simulink model "SSN_39busRT_Ctrl_4WT_19B"  (R2021a)
settings: Solver=ode3  StartTime=0.0  StopTime=10  FixedStep=Ts  MaxStep=1/60  RelTol=1e-2  AbsTol=1e-1
PreLoadFcn:
  | Ts=2.50e-6; ssn_ieee39_params; load('Pwf.mat');
InitFcn:
  | Ts=2.50e-6; ssn_ieee39_params; load('Pwf.mat');
values from neighbouring files (symbols this model uses):
  f = 50    [ssn_ieee39_params_ctrl.m]
  fNom = f    (= 60)    [ssn_ieee39_params_ctrl.m]
  ILR = 5.02    [ssn_ieee39_params_ctrl.m]
  IQMIN = 0.1    [ssn_ieee39_params_ctrl.m]
  ISCLIM = 1    [ssn_ieee39_params_ctrl.m]
  ITFpu = 1.10    (= 1.1)    [ssn_ieee39_params_ctrl.m]
  K = 1    [ssn_ieee39_params_ctrl.m]
  K1 = 1    [ssn_ieee39_params_ctrl.m]
  K2 = 2    [ssn_ieee39_params_ctrl.m]
  KCL = 1.04    [ssn_ieee39_params_ctrl.m]
  KFB = 0    [ssn_ieee39_params_ctrl.m]
  KFF = 1    [ssn_ieee39_params_ctrl.m]
  KFIX = 1    [ssn_ieee39_params_ctrl.m]
  KG = 1    [ssn_ieee39_params_ctrl.m]
  KIA = 59.91    [ssn_ieee39_params_ctrl.m]
  KIOEX = 0.0303    [ssn_ieee39_params_ctrl.m]
  KIUEX = 0.0303    [ssn_ieee39_params_ctrl.m]
  KIUOEX = 1    [ssn_ieee39_params_ctrl.m]
  KIUUEX = 1    [ssn_ieee39_params_ctrl.m]
  KLR = 22.47    [ssn_ieee39_params_ctrl.m]
  KM = 1    [ssn_ieee39_params_ctrl.m]
  KOEL = 0.24    [ssn_ieee39_params_ctrl.m]
  Kp = 1    [ssn_ieee39_params_ctrl.m]
  KPA = 30    [ssn_ieee39_params_ctrl.m]
  KPOEL = 1    [ssn_ieee39_params_ctrl.m]
  KPOEX = 0    [ssn_ieee39_params_ctrl.m]
  KPUEX = 0    [ssn_ieee39_params_ctrl.m]
  KSCALE = 0.319    [ssn_ieee39_params_ctrl.m]
  KUF = 0    [ssn_ieee39_params_ctrl.m]
  KUI = 0.001    [ssn_ieee39_params_ctrl.m]
  KUL = 0.24    [ssn_ieee39_params_ctrl.m]
  s = 10    [ssn_ieee39_params_ctrl.m]
  TA = 0.01    [ssn_ieee39_params_ctrl.m]
  Tadj = 0    [ssn_ieee39_params_ctrl.m]
  taps = [1 1 1.07 1.07 1.009 1.025 1 1.025 1.025 1.025]*1    [ssn_ieee39_params_ctrl.m]
  TF = 0.02    [ssn_ieee39_params_ctrl.m]
  TG = 0.024    [ssn_ieee39_params_ctrl.m]
  TINV = 0    [ssn_ieee39_params_ctrl.m]
  TIT = 0.1    [ssn_ieee39_params_ctrl.m]
  TL_10_11_len = 14    [ssn_ieee39_params_ctrl.m]
  TL_10_13_len = 14    [ssn_ieee39_params_ctrl.m]
  TL_13_14_len = 32    [ssn_ieee39_params_ctrl.m]
  TL_14_15_len = 70    [ssn_ieee39_params_ctrl.m]
  TL_15_16_len = 31.5    [ssn_ieee39_params_ctrl.m]
  TL_16_17_len = 26    [ssn_ieee39_params_ctrl.m]
  TL_16_19_len = 61    [ssn_ieee39_params_ctrl.m]
  TL_16_21_len = 46    [ssn_ieee39_params_ctrl.m]
  TL_16_24_len = 15    [ssn_ieee39_params_ctrl.m]
  TL_17_18_len = 26    [ssn_ieee39_params_ctrl.m]
  TL_17_27_len = 59    [ssn_ieee39_params_ctrl.m]
  TL_1_2_len = 134    [ssn_ieee39_params_ctrl.m]
  TL_1_39_len = 105    [ssn_ieee39_params_ctrl.m]
  TL_21_22_len = 47    [ssn_ieee39_params_ctrl.m]
  TL_22_23_len = 33    [ssn_ieee39_params_ctrl.m]
  TL_24_23_len = 88    [ssn_ieee39_params_ctrl.m]
  TL_25_26_len = 101    [ssn_ieee39_params_ctrl.m]
  TL_26_27_len = 46.5    [ssn_ieee39_params_ctrl.m]
  TL_26_28_len = 151    [ssn_ieee39_params_ctrl.m]
  TL_26_29_len = 200    [ssn_ieee39_params_ctrl.m]
  TL_28_29_len = 48    [ssn_ieee39_params_ctrl.m]
  TL_2_25_len = 28    [ssn_ieee39_params_ctrl.m]
  TL_2_2_len = 49    [ssn_ieee39_params_ctrl.m]
  TL_3_18_len = 42    [ssn_ieee39_params_ctrl.m]
  TL_3_4_len = 53    [ssn_ieee39_params_ctrl.m]
  TL_4_14_len = 33    [ssn_ieee39_params_ctrl.m]
  TL_4_5_len = 32.5    [ssn_ieee39_params_ctrl.m]
  TL_5_6_len = 14    [ssn_ieee39_params_ctrl.m]
  TL_5_8_len = 32    [ssn_ieee39_params_ctrl.m]
  TL_6_11_len = 26.5    [ssn_ieee39_params_ctrl.m]
  TL_6_7_len = 25.5    [ssn_ieee39_params_ctrl.m]
  TL_7_8_len = 15    [ssn_ieee39_params_ctrl.m]
  TL_8_9_len = 93    [ssn_ieee39_params_ctrl.m]
  TL_9_39_len = 136    [ssn_ieee39_params_ctrl.m]
  TOEL = 5.00    (= 5)    [ssn_ieee39_params_ctrl.m]
  TQREF = 0    [ssn_ieee39_params_ctrl.m]
  TQSCL = 0.012    [ssn_ieee39_params_ctrl.m]
  Ts_PMU = 1/1000    (= 0.001)    [ssn_ieee39_params_ctrl.m]
  TU1 = 0    [ssn_ieee39_params_ctrl.m]
  TU2 = 0    [ssn_ieee39_params_ctrl.m]
  TU3 = 0    [ssn_ieee39_params_ctrl.m]
  TU4 = 0    [ssn_ieee39_params_ctrl.m]
  TUL = 0    [ssn_ieee39_params_ctrl.m]
  TUP = 0.050    (= 0.05)    [ssn_ieee39_params_ctrl.m]
  TUQ = .005    (= 0.005)    [ssn_ieee39_params_ctrl.m]
  TUV = 0.2    [ssn_ieee39_params_ctrl.m]
  VAAMAX = VAMAX    (= 7.05)    [ssn_ieee39_params_ctrl.m]
  VAMAX = 7.05    [ssn_ieee39_params_ctrl.m]
  VAMIN = -6.11    [ssn_ieee39_params_ctrl.m]
  VBMAX = 999    [ssn_ieee39_params_ctrl.m]
  VF = 0    [ssn_ieee39_params_ctrl.m]
  VFB = 0    [ssn_ieee39_params_ctrl.m]
  VMMAX = 7.05    [ssn_ieee39_params_ctrl.m]
  VMMIN = -6.11    [ssn_ieee39_params_ctrl.m]
  VOELmax1 = 0.2353    [ssn_ieee39_params_ctrl.m]
  VOELmax2 = 0.0    (= 0)    [ssn_ieee39_params_ctrl.m]
  VOELmin1 = -0.24    [ssn_ieee39_params_ctrl.m]
  VOELmin2 = -1.0    (= -1)    [ssn_ieee39_params_ctrl.m]
  VRMAX = 7.05    [ssn_ieee39_params_ctrl.m]
  VRMIN = -6.11    [ssn_ieee39_params_ctrl.m]
  VSCLmax = 0.20    (= 0.2)    [ssn_ieee39_params_ctrl.m]
  VSCLmin = -0.10    (= -0.1)    [ssn_ieee39_params_ctrl.m]
  VUELmax1 = 1    [ssn_ieee39_params_ctrl.m]
  VUELmax2 = 1    [ssn_ieee39_params_ctrl.m]
  VUELmin1 = -1    [ssn_ieee39_params_ctrl.m]
  VUELmin2 = -1    [ssn_ieee39_params_ctrl.m]
  VUImax = 1    [ssn_ieee39_params_ctrl.m]
  VUImin = -1    [ssn_ieee39_params_ctrl.m]
undefined symbols (not defined in the file or in its folder): another_event_name, D1, Delta, DiscIntNeverNeededParam, find_system, MOV_segment9, my_event_name, powergui, Pw1, Pw2, Pw3, Pw4, vNomHV
libraries: powerlib_extras x162, spsThreePhaseVIMeasurementLib x55, spsCurrentMeasurementLib x52, simulink_extras x44, slpidlib x40, op_dpl_lib x36, spsST2AModel x20, spsThreePhaseParallelRLCLoadLib x20, spsThreePhaseTransformerTwoWindingsLib x17, spsControlledVoltageSourceLib x16, spsVoltageMeasurementLib x12, spsSynchronousMachinepuStandardLib x10
(part 14 of 19)

== system SSN_39busRT_Ctrl_4WT_19B/SM_master/4 WT/SS_windfarm3to4/Wind Farm (DFIG Type)/Wind Turbine Doubly-Fed Induction Generator (Average Model)1 ==
  Wind Power : Inport
  Asynchronous Machine pu Units1 : spsAsynchronousMachinepuUnitsLib/Asynchronous Machine pu Units  RotorType=Wound  PresetModel=No  MechanicalLoad=Torque Tm  ShowDetailedParameters=on  ReferenceFrame=Rotor  Units=pu  MeasurementBus=off  NominalParameters=[ Pnom*NumberOfUnits Vnom Fnom ]  VoltageRatio=1  Stator=[ Rs Lls]  Rotor=[ Rr Llr]  Cage1=[0.01909 0.0397]  Cage2=[0.01909 0.0397]  Lm=Lm  Mechanical=[H F p]  PolePairs=3  InitialConditions=[-4.81362e-32 0 0.00115467 0.00115467 0.00115467 -120.432 119.568 -0.43182]  SimulateSaturation=off  Saturation="[0.212,0.4201,0.8125,1.0979,1.4799,2.2457,3.2586,4.5763,6.4763 ;   0.5,0.7,0.9,1,1.1,1.2 ,1.3,1.4,1.5]"  LoadFlowParameters=0  TsPowergui=0  TsBlock=-1  IterativeModel=Forward Euler  IterativeDiscreteModel=Trapezoidal non iterative  Pmec=0
      settings: SourceProductBaseCode=PS
  Average_VSC : Subsystem  mask(Average Voltage Source converter){Ts=Ts_Power}
      mask prompts: Ts "Sample time"
  Average_VSC1 : Subsystem  mask(Average Voltage Source converter){Ts=Ts_Power}
      mask prompts: Ts "Sample time"
  B1 : spsThreePhaseVIMeasurementLib/Three-Phase V-I Measurement  VoltageMeasurement=phase-to-ground  SetLabelV=off  LabelV=Vabc_B1  Vpu=on  VpuLL=off  CurrentMeasurement=yes  SetLabelI=off  LabelI=Iabc_Beol  Ipu=on  Pbase=Pnom*NumberOfUnits  Vbase=Vnom  OutputType=Complex  PhasorSimulation=off  PSBequivalent=0
  Bus Selector : BusSelector  OutputSignals=Mechanical.Rotor speed (wm),Mechanical.Rotor angle thetam (rad),Mechanical.Electromagnetic torque Te (pu)
  C2 : spsSeriesRLCBranchLib/Series RLC Branch  LConnTagsString=__new0  RConnTagsString=__new0  BranchType=C  Resistance=1.0  Inductance=1.0  SetiL0=off  InitialCurrent=0  Capacitance=C_DClink*NumberOfUnits  Setx0=off  InitialVoltage=0  Measurements=Branch voltage
  Control System_average : Subsystem  mask{Pmax=0.5, Vdc_nom=Vdc_nom*1.2, capacitor=C_DClink*NumberOfUnits, speed_ABCD=[0.7 0.71 1.2 1.21], power_C=power_C, pitch_gain=500, pitch_max=45, pitch_rate=2, Kpi_Q=[0.05 5], Kpi_dc_reg=[0.002 0.05], Kpi_grid_side_cur_reg=[2.5 500], Kpi_rotor_side_cur_reg=[0.3 8], Q_slew_rate=100, torque_slew_rate=1, current_slew_rate=200, Ts=Ts_Power, Ts_Control=Ts_Control}
      mask prompts: Pmax "Converter maximum power (p.u.):"; Vdc_nom "Nominal DC bus voltage (V):"; capacitor "DC bus capacitor (F):"; speed_ABCD "Tracking characteristic speeds: [speed_A(pu) ... speed_D(pu)]"; power_C "Power at point C (pu/mechanical power):"; pitch_gain "Pitch angle controller gain [Kp]:"; pitch_max "Maximum pitch angle (deg):"; pitch_rate "Maximum rate of change of pitch angle (deg/s):"; Kpi_Q "Reactive power regulator gains: [Kp Ki]"; Kpi_dc_reg "DC bus voltage regulator gains: [Kp Ki]"; Kpi_grid_side_cur_reg "Grid-side converter current regulator gains: [Kp Ki]"; Kpi_rotor_side_cur_reg "Rotor-side converter current regulator gains: [Kp Ki]"; Q_slew_rate "Maximum rate of change of reference reactive power (p.u./s):"; torque_slew_rate "Maximum rate of change of reference torque (p.u./s):"; current_slew_rate "Maximum rate of change of converter  reference currents (p.u./s):"; Ts "Sample time"; Ts_Control "Sample time control"
      mask init: same as SSN_39busRT_Ctrl_4WT_19B/SM_master/4 WT/SS_windfarm1to2/Wind Farm (DFIG Type)/Wind Turbine Doubly-Fed Induction Generator (Average Model)1/Control System_average
  Data acquisition electrical : Subsystem
  "Iq_ref (pu) " : Constant  Value=0
  "Qref (pu) " : Constant  Value=0
  Subsystem : Subsystem
  Subsystem1 : Subsystem
  Subsystem2 : Subsystem
  Vc1 : spsVoltageMeasurementLib/Voltage Measurement  PhasorSimulation=off  OutputType=Complex  PSBequivalent=0
  Wind Turbine v : Subsystem  mask{Pnom=Pmec*NumberOfUnits, Pelec_base=Pnom*NumberOfUnits, wind_base=11, P_wind_base=power_C, speed_nom=speed_C, pitch_angle=0, c1_c6=[0.51763          116          0.4            5           21     0.006795], cp_nom=0.48, lambda_nom=8.1}
      mask prompts: Pnom "Nominal mechanical output power(W):"; Pelec_base "Base power of the electrical genera(VA):"; wind_base "Base wind speed(m/s):"; P_wind_base "Maximum powe at base wind speed(pu of nominal mechanical power):"; speed_nom "Base rotational speed(p.u. of base generator speed):"; pitch_angle "Pitch angle beta to display wind-turbine power"
      mask init:
      | c1=c1_c6(1);c2=c1_c6(2);c3=c1_c6(3);c4=c1_c6(4);c5=c1_c6(5);c6=c1_c6(6);
      | power_initmask();
      mask DialogControl DisplayTurbChar Prompt: Display wind turbine power characteristics
      mask DialogControl DisplayTurbChar Callback: WindTurbinePlot(gcb)
  "choke " : spsThreePhaseSeriesRLCBranchLib/Three-Phase Series RLC Branch  LConnTagsString=A|B|C  RConnTagsString=A|B|C  BranchType=RL  Resistance=R_RL*Vnom^2/(Pnom*NumberOfUnits)  Inductance=L_RL*Vnom^2/(Pnom*NumberOfUnits)/(2*pi*Fnom)  Capacitance=1.0  Measurements=None
  A : PMIOPort  Side=Left
  B : PMIOPort  Port=2  Side=Left
  C : PMIOPort  Port=3  Side=Left
  meas_elec : Outport
  wires:
  "Iq_ref (pu) "/1 -> Control System_average/3(Iq_grid_conv_ref)
  "Qref (pu) "/1 -> Control System_average/2(Q_ref)
  [Vabc_B1] -> Control System_average/1(Vabc_B1)
  B1/1 -> [Vabc_B1]
  B1/2 -> [Iabc_B1]
  Subsystem2/1(IabcPU) -> [Iabc_stator]
  [wr] -> Control System_average/4(wr)
  [Iabc_grid_conv] -> Control System_average/5(Iabc_grid_conv)
  [Iabc_stator] -> Control System_average/6(Iabc_stator)
  [Iabc_rotor] -> Control System_average/7(Iabc_rotor)
  [Q_B1] -> Control System_average/8(Q_B1)
  Control System_average/3(Theta_Freq) -> [Theta_Freq]
  Control System_average/4(Pitch_angle) -> [Beta]
  [Vabc_B1] -> Data acquisition electrical/1(Vabc_B1)
  Data acquisition electrical/1(meas) -> meas_elec/1
  Data acquisition electrical/2(Q_B1) -> [Q_B1]
  [Iabc_B1] -> Data acquisition electrical/2(Iabc_B1)
  [Theta_Freq] -> Data acquisition electrical/3(Theta_Freq)
  [angle_rotor] -> Control System_average/9(angle_rotor)
  [Vdc] -> Control System_average/10(Vdc)
  Subsystem/1(IabcPU) -> [Iabc_grid_conv]
  Subsystem1/1(IabcPU) -> [Iabc_rotor]
  [Tm] -> Asynchronous Machine pu Units1/1
  Bus Selector/1 -> [wr]  "<Rotor speed (wm)>"
  Bus Selector/2 -> [angle_rotor]  "<Rotor angle thetam (rad)>"
  Asynchronous Machine pu Units1/1 -> Bus Selector/1
  [Vdc] -> Data acquisition electrical/4(Vdc)
  Vc1/1 -> [Vdc]
  Control System_average/1(Uref_grid_conv) -> Average_VSC/1(Uref)
  Control System_average/2(Uref_rotor_conv) -> Average_VSC1/1(Uref)
  Bus Selector/3 -> [Tem]  "<Electromagnetic torque Te (pu)>"
  [wr] -> Wind Turbine v/1(Generator speed (pu))
  Wind Power/1 -> Wind Turbine v/2(Wind Power)  "Pwind_pu"
  Wind Turbine v/1(Tm (pu)) -> [Tm]
  connections:
  "choke "/LConn1 -- Subsystem2/LConn1 -- B1/RConn1
  "choke "/LConn2 -- Subsystem2/LConn2 -- B1/RConn2
  "choke "/LConn3 -- Subsystem2/LConn3 -- B1/RConn3
  C/RConn1 -- B1/LConn3
  B/RConn1 -- B1/LConn2
  A/RConn1 -- B1/LConn1
  "choke "/RConn1 -- Subsystem/LConn1
  "choke "/RConn2 -- Subsystem/LConn2
  "choke "/RConn3 -- Subsystem/LConn3
  Subsystem2/RConn1 -- Asynchronous Machine pu Units1/LConn1
  Subsystem2/RConn2 -- Asynchronous Machine pu Units1/LConn2
  Subsystem2/RConn3 -- Asynchronous Machine pu Units1/LConn3
  Subsystem1/RConn1 -- Asynchronous Machine pu Units1/RConn1
  Subsystem1/RConn2 -- Asynchronous Machine pu Units1/RConn2
  Subsystem1/RConn3 -- Asynchronous Machine pu Units1/RConn3
  Average_VSC1/RConn1 -- C2/LConn1 -- Average_VSC/RConn1 -- Vc1/LConn1
  Average_VSC1/RConn2 -- C2/RConn1 -- Average_VSC/RConn2 -- Vc1/LConn2
  Subsystem1/LConn1 -- Average_VSC1/LConn1
  Subsystem1/LConn2 -- Average_VSC1/LConn2
  Subsystem1/LConn3 -- Average_VSC1/LConn3
  Subsystem/RConn1 -- Average_VSC/LConn1
  Subsystem/RConn2 -- Average_VSC/LConn2
  Subsystem/RConn3 -- Average_VSC/LConn3

== system SSN_39busRT_Ctrl_4WT_19B/SM_master/4 WT/SS_windfarm3to4/Wind Farm (DFIG Type)2/Wind Turbine Doubly-Fed Induction Generator (Average Model)1 ==
  Wind Power : Inport
  Asynchronous Machine pu Units1 : spsAsynchronousMachinepuUnitsLib/Asynchronous Machine pu Units  RotorType=Wound  PresetModel=No  MechanicalLoad=Torque Tm  ShowDetailedParameters=on  ReferenceFrame=Rotor  Units=pu  MeasurementBus=off  NominalParameters=[ Pnom*NumberOfUnits Vnom Fnom ]  VoltageRatio=1  Stator=[ Rs Lls]  Rotor=[ Rr Llr]  Cage1=[0.01909 0.0397]  Cage2=[0.01909 0.0397]  Lm=Lm  Mechanical=[H F p]  PolePairs=3  InitialConditions=[-4.81362e-32 0 0.00115467 0.00115467 0.00115467 -120.432 119.568 -0.43182]  SimulateSaturation=off  Saturation="[0.212,0.4201,0.8125,1.0979,1.4799,2.2457,3.2586,4.5763,6.4763 ;   0.5,0.7,0.9,1,1.1,1.2 ,1.3,1.4,1.5]"  LoadFlowParameters=0  TsPowergui=0  TsBlock=-1  IterativeModel=Forward Euler  IterativeDiscreteModel=Trapezoidal non iterative  Pmec=0
      settings: SourceProductBaseCode=PS
  Average_VSC : Subsystem  mask(Average Voltage Source converter){Ts=Ts_Power}
      mask prompts: Ts "Sample time"
  Average_VSC1 : Subsystem  mask(Average Voltage Source converter){Ts=Ts_Power}
      mask prompts: Ts "Sample time"
  B1 : spsThreePhaseVIMeasurementLib/Three-Phase V-I Measurement  VoltageMeasurement=phase-to-ground  SetLabelV=off  LabelV=Vabc_B1  Vpu=on  VpuLL=off  CurrentMeasurement=yes  SetLabelI=off  LabelI=Iabc_Beol  Ipu=on  Pbase=Pnom*NumberOfUnits  Vbase=Vnom  OutputType=Complex  PhasorSimulation=off  PSBequivalent=0
  Bus Selector : BusSelector  OutputSignals=Mechanical.Rotor speed (wm),Mechanical.Rotor angle thetam (rad),Mechanical.Electromagnetic torque Te (pu)
  C2 : spsSeriesRLCBranchLib/Series RLC Branch  LConnTagsString=__new0  RConnTagsString=__new0  BranchType=C  Resistance=1.0  Inductance=1.0  SetiL0=off  InitialCurrent=0  Capacitance=C_DClink*NumberOfUnits  Setx0=off  InitialVoltage=0  Measurements=Branch voltage
  Control System_average : Subsystem  mask{Pmax=0.5, Vdc_nom=Vdc_nom*1.2, capacitor=C_DClink*NumberOfUnits, speed_ABCD=[0.7 0.71 1.2 1.21], power_C=power_C, pitch_gain=500, pitch_max=45, pitch_rate=2, Kpi_Q=[0.05 5], Kpi_dc_reg=[0.002 0.05], Kpi_grid_side_cur_reg=[2.5 500], Kpi_rotor_side_cur_reg=[0.3 8], Q_slew_rate=100, torque_slew_rate=1, current_slew_rate=200, Ts=Ts_Power, Ts_Control=Ts_Control}
      mask prompts: Pmax "Converter maximum power (p.u.):"; Vdc_nom "Nominal DC bus voltage (V):"; capacitor "DC bus capacitor (F):"; speed_ABCD "Tracking characteristic speeds: [speed_A(pu) ... speed_D(pu)]"; power_C "Power at point C (pu/mechanical power):"; pitch_gain "Pitch angle controller gain [Kp]:"; pitch_max "Maximum pitch angle (deg):"; pitch_rate "Maximum rate of change of pitch angle (deg/s):"; Kpi_Q "Reactive power regulator gains: [Kp Ki]"; Kpi_dc_reg "DC bus voltage regulator gains: [Kp Ki]"; Kpi_grid_side_cur_reg "Grid-side converter current regulator gains: [Kp Ki]"; Kpi_rotor_side_cur_reg "Rotor-side converter current regulator gains: [Kp Ki]"; Q_slew_rate "Maximum rate of change of reference reactive power (p.u./s):"; torque_slew_rate "Maximum rate of change of reference torque (p.u./s):"; current_slew_rate "Maximum rate of change of converter  reference currents (p.u./s):"; Ts "Sample time"; Ts_Control "Sample time control"
      mask init: same as SSN_39busRT_Ctrl_4WT_19B/SM_master/4 WT/SS_windfarm1to2/Wind Farm (DFIG Type)/Wind Turbine Doubly-Fed Induction Generator (Average Model)1/Control System_average
  Data acquisition electrical : Subsystem
  "Iq_ref (pu) " : Constant  Value=0
  "Qref (pu) " : Constant  Value=0
  Subsystem : Subsystem
  Subsystem1 : Subsystem
  Subsystem2 : Subsystem
  Vc1 : spsVoltageMeasurementLib/Voltage Measurement  PhasorSimulation=off  OutputType=Complex  PSBequivalent=0
  Wind Turbine v : Subsystem  mask{Pnom=Pmec*NumberOfUnits, Pelec_base=Pnom*NumberOfUnits, wind_base=11, P_wind_base=power_C, speed_nom=speed_C, pitch_angle=0, c1_c6=[0.51763          116          0.4            5           21     0.006795], cp_nom=0.48, lambda_nom=8.1}
      mask prompts: Pnom "Nominal mechanical output power(W):"; Pelec_base "Base power of the electrical genera(VA):"; wind_base "Base wind speed(m/s):"; P_wind_base "Maximum powe at base wind speed(pu of nominal mechanical power):"; speed_nom "Base rotational speed(p.u. of base generator speed):"; pitch_angle "Pitch angle beta to display wind-turbine power"
      mask init:
      | c1=c1_c6(1);c2=c1_c6(2);c3=c1_c6(3);c4=c1_c6(4);c5=c1_c6(5);c6=c1_c6(6);
      | power_initmask();
      mask DialogControl DisplayTurbChar Prompt: Display wind turbine power characteristics
      mask DialogControl DisplayTurbChar Callback: WindTurbinePlot(gcb)
  "choke " : spsThreePhaseSeriesRLCBranchLib/Three-Phase Series RLC Branch  LConnTagsString=A|B|C  RConnTagsString=A|B|C  BranchType=RL  Resistance=R_RL*Vnom^2/(Pnom*NumberOfUnits)  Inductance=L_RL*Vnom^2/(Pnom*NumberOfUnits)/(2*pi*Fnom)  Capacitance=1.0  Measurements=None
  A : PMIOPort  Side=Left
  B : PMIOPort  Port=2  Side=Left
  C : PMIOPort  Port=3  Side=Left
  meas_elec : Outport
  wires:
  Wind Turbine v/1(Tm (pu)) -> [Tm]
  Wind Power/1 -> Wind Turbine v/2(Wind Power)  "Pwind_pu"
  [wr] -> Wind Turbine v/1(Generator speed (pu))
  Bus Selector/3 -> [Tem]  "<Electromagnetic torque Te (pu)>"
  Control System_average/2(Uref_rotor_conv) -> Average_VSC1/1(Uref)
  Control System_average/1(Uref_grid_conv) -> Average_VSC/1(Uref)
  Vc1/1 -> [Vdc]
  [Vdc] -> Data acquisition electrical/4(Vdc)
  Asynchronous Machine pu Units1/1 -> Bus Selector/1
  Bus Selector/2 -> [angle_rotor]  "<Rotor angle thetam (rad)>"
  Bus Selector/1 -> [wr]  "<Rotor speed (wm)>"
  [Tm] -> Asynchronous Machine pu Units1/1
  Subsystem1/1(IabcPU) -> [Iabc_rotor]
  Subsystem/1(IabcPU) -> [Iabc_grid_conv]
  [Vdc] -> Control System_average/10(Vdc)
  [angle_rotor] -> Control System_average/9(angle_rotor)
  [Theta_Freq] -> Data acquisition electrical/3(Theta_Freq)
  [Iabc_B1] -> Data acquisition electrical/2(Iabc_B1)
  Data acquisition electrical/2(Q_B1) -> [Q_B1]
  Data acquisition electrical/1(meas) -> meas_elec/1
  [Vabc_B1] -> Data acquisition electrical/1(Vabc_B1)
  Control System_average/4(Pitch_angle) -> [Beta]
  Control System_average/3(Theta_Freq) -> [Theta_Freq]
  [Q_B1] -> Control System_average/8(Q_B1)
  [Iabc_rotor] -> Control System_average/7(Iabc_rotor)
  [Iabc_stator] -> Control System_average/6(Iabc_stator)
  [Iabc_grid_conv] -> Control System_average/5(Iabc_grid_conv)
  [wr] -> Control System_average/4(wr)
  Subsystem2/1(IabcPU) -> [Iabc_stator]
  B1/2 -> [Iabc_B1]
  B1/1 -> [Vabc_B1]
  [Vabc_B1] -> Control System_average/1(Vabc_B1)
  "Qref (pu) "/1 -> Control System_average/2(Q_ref)
  "Iq_ref (pu) "/1 -> Control System_average/3(Iq_grid_conv_ref)
  connections:
  Subsystem/RConn3 -- Average_VSC/LConn3
  Subsystem/RConn2 -- Average_VSC/LConn2
  Subsystem/RConn1 -- Average_VSC/LConn1
  Subsystem1/LConn3 -- Average_VSC1/LConn3
  Subsystem1/LConn2 -- Average_VSC1/LConn2
  Subsystem1/LConn1 -- Average_VSC1/LConn1
  Vc1/LConn2 -- Average_VSC/RConn2 -- C2/RConn1 -- Average_VSC1/RConn2
  Vc1/LConn1 -- Average_VSC/RConn1 -- C2/LConn1 -- Average_VSC1/RConn1
  Subsystem1/RConn3 -- Asynchronous Machine pu Units1/RConn3
  Subsystem1/RConn2 -- Asynchronous Machine pu Units1/RConn2
  Subsystem1/RConn1 -- Asynchronous Machine pu Units1/RConn1
  Subsystem2/RConn3 -- Asynchronous Machine pu Units1/LConn3
  Subsystem2/RConn2 -- Asynchronous Machine pu Units1/LConn2
  Subsystem2/RConn1 -- Asynchronous Machine pu Units1/LConn1
  "choke "/RConn3 -- Subsystem/LConn3
  "choke "/RConn2 -- Subsystem/LConn2
  "choke "/RConn1 -- Subsystem/LConn1
  A/RConn1 -- B1/LConn1
  B/RConn1 -- B1/LConn2
  C/RConn1 -- B1/LConn3
  B1/RConn3 -- Subsystem2/LConn3 -- "choke "/LConn3
  B1/RConn2 -- Subsystem2/LConn2 -- "choke "/LConn2
  B1/RConn1 -- Subsystem2/LConn1 -- "choke "/LConn1

== system SSN_39busRT_Ctrl_4WT_19B/SM_master/4 WT/controlWt/Subsystem/Wind speed data ==
  Ctr12 : Inport
  Ctr34 : Inport  Port=2
  Clock : Inport  Port=3
  1-D Lookup Table : Lookup_n-D  NumberOfTableDimensions=1  BreakpointsForDimension1=[1:3600]  Table=Pw1  InterpMethod=Flat  ExtrapMethod=Cubic spline  DiagnosticForOutOfRangeInput=Error  InternalRulePriority=Speed  RndMeth=Simplest  InputSameDT=on
  1-D Lookup Table1 : Lookup_n-D  NumberOfTableDimensions=1  BreakpointsForDimension1=[1:3600]  Table=Pw3  InterpMethod=Flat  ExtrapMethod=Cubic spline  DiagnosticForOutOfRangeInput=Error  InternalRulePriority=Speed  RndMeth=Simplest  InputSameDT=on
  1-D Lookup Table2 : Lookup_n-D  NumberOfTableDimensions=1  BreakpointsForDimension1=[1:3600]  Table=Pw2  InterpMethod=Flat  ExtrapMethod=Cubic spline  DiagnosticForOutOfRangeInput=Error  InternalRulePriority=Speed  RndMeth=Simplest  InputSameDT=on
  1-D Lookup Table3 : Lookup_n-D  NumberOfTableDimensions=1  BreakpointsForDimension1=[1:3600]  Table=Pw4  InterpMethod=Flat  ExtrapMethod=Cubic spline  DiagnosticForOutOfRangeInput=Error  InternalRulePriority=Speed  RndMeth=Simplest  InputSameDT=on
  Constant : Constant
  Constant1 : Constant  Value=0.8206
  Constant2 : Constant  Value=0.8268
  Constant3 : Constant  Value=0.7
  Constant4 : Constant  Value=0.7303
  Mux{1..5,15} (6 alike) : Mux  Inputs=2
  Rounding Function : Rounding
  Sum : Sum  Inputs=|++
  Terminator : Terminator
  Terminator1 : Terminator
  wf12 : Outport
  wf34 : Outport  Port=2
  wires:
  Ctr12/1 -> Mux15/2
  Mux15/1 -> wf12/1
  Constant/1 -> Sum/2
  Clock/1 -> Rounding Function/1
  1-D Lookup Table/1 -> Mux2/1
  Ctr34/1 -> Mux1/2
  Mux1/1 -> wf34/1
  1-D Lookup Table2/1 -> Mux2/2
  Sum/1 -> 1-D Lookup Table3/1, 1-D Lookup Table1/1, 1-D Lookup Table2/1, 1-D Lookup Table/1
  1-D Lookup Table1/1 -> Mux3/1
  1-D Lookup Table3/1 -> Mux3/2
  Mux3/1 -> Mux1/1
  Rounding Function/1 -> Sum/1
  Constant1/1 -> Mux4/1
  Constant2/1 -> Mux4/2
  Mux2/1 -> Mux15/1
  Constant3/1 -> Mux5/1
  Constant4/1 -> Mux5/2
  Mux5/1 -> Terminator1/1
  Mux4/1 -> Terminator/1

== system SSN_39busRT_Ctrl_4WT_19B/SM_master/4 WT/SS_windfarm1to2/Wind Farm (DFIG Type)/Wind Turbine Doubly-Fed Induction Generator (Average Model)1/Average_VSC ==
  Uref : Inport
  Converter_model : Subsystem
  Demux : Demux  Outputs=2
  Ia_meas : spsCurrentMeasurementLib/Current Measurement  PhasorSimulation=off  OutputType=Complex  PSBequivalent=0
  Ic_meas : spsCurrentMeasurementLib/Current Measurement  PhasorSimulation=off  OutputType=Complex  PSBequivalent=0
  Idc : spsControlledCurrentSourceLib/Controlled Current Source  Initialize=on  Source_Type=AC  Amplitude=0  Phase=0  Frequency=0  Measurements=None
  Mux : Mux  Inputs=2
  Vab : spsControlledVoltageSourceLib/Controlled Voltage Source  Initialize=on  Source_Type=AC  Amplitude=0  Phase=0  Frequency=0  Measurements=None
  Vbc : spsControlledVoltageSourceLib/Controlled Voltage Source  Initialize=on  Source_Type=AC  Amplitude=0  Phase=0  Frequency=0  Measurements=None
  Vdc_meas : spsVoltageMeasurementLib/Voltage Measurement  PhasorSimulation=off  OutputType=Complex  PSBequivalent=0
  A : PMIOPort  Side=Left
  B : PMIOPort  Port=2  Side=Left
  C : PMIOPort  Port=3  Side=Left
  + : PMIOPort  Port=4  Side=Right
  - : PMIOPort  Port=5  Side=Right
  wires:
  Converter_model/2(Vab_Vbc) -> Demux/1
  Converter_model/1(Idc) -> Idc/1  "Idc"
  Mux/1 -> Converter_model/1(Ia_Ic)
  Vdc_meas/1 -> Converter_model/2(Vdc)
  Uref/1 -> Converter_model/3(Uref)
  Ic_meas/1 -> Mux/2  "Ic"
  Ia_meas/1 -> Mux/1  "Ia"
  Demux/1 -> Vab/1  "Vab"
  Demux/2 -> Vbc/1  "Vbc"
  connections:
  Idc/LConn1 -- -/RConn1 -- Vdc_meas/LConn1
  Idc/RConn1 -- +/RConn1 -- Vdc_meas/LConn2
  C/RConn1 -- Ic_meas/LConn1
  A/RConn1 -- Ia_meas/LConn1
  Ia_meas/RConn1 -- Vab/LConn1
  B/RConn1 -- Vbc/LConn1 -- Vab/RConn1
  Vbc/RConn1 -- Ic_meas/RConn1

== system SSN_39busRT_Ctrl_4WT_19B/SM_master/4 WT/SS_windfarm1to2/Wind Farm (DFIG Type)/Wind Turbine Doubly-Fed Induction Generator (Average Model)1/Average_VSC1 ==
  Uref : Inport
  Converter_model : Subsystem
  Demux : Demux  Outputs=2
  Ia_meas : spsCurrentMeasurementLib/Current Measurement  PhasorSimulation=off  OutputType=Complex  PSBequivalent=0
  Ic_meas : spsCurrentMeasurementLib/Current Measurement  PhasorSimulation=off  OutputType=Complex  PSBequivalent=0
  Idc : spsControlledCurrentSourceLib/Controlled Current Source  Initialize=on  Source_Type=AC  Amplitude=0  Phase=0  Frequency=0  Measurements=None
  Mux : Mux  Inputs=2
  Vab : spsControlledVoltageSourceLib/Controlled Voltage Source  Initialize=on  Source_Type=AC  Amplitude=0  Phase=0  Frequency=0  Measurements=None
  Vbc : spsControlledVoltageSourceLib/Controlled Voltage Source  Initialize=on  Source_Type=AC  Amplitude=0  Phase=0  Frequency=0  Measurements=None
  Vdc_meas : spsVoltageMeasurementLib/Voltage Measurement  PhasorSimulation=off  OutputType=Complex  PSBequivalent=0
  A : PMIOPort  Side=Left
  B : PMIOPort  Port=2  Side=Left
  C : PMIOPort  Port=3  Side=Left
  + : PMIOPort  Port=4  Side=Right
  - : PMIOPort  Port=5  Side=Right
  wires:
  Converter_model/2(Vab_Vbc) -> Demux/1
  Converter_model/1(Idc) -> Idc/1  "Idc"
  Mux/1 -> Converter_model/1(Ia_Ic)
  Vdc_meas/1 -> Converter_model/2(Vdc)
  Uref/1 -> Converter_model/3(Uref)
  Ic_meas/1 -> Mux/2  "Ic"
  Ia_meas/1 -> Mux/1  "Ia"
  Demux/1 -> Vab/1  "Vab"
  Demux/2 -> Vbc/1  "Vbc"
  connections:
  Idc/LConn1 -- -/RConn1 -- Vdc_meas/LConn1
  Idc/RConn1 -- +/RConn1 -- Vdc_meas/LConn2
  C/RConn1 -- Ic_meas/LConn1
  A/RConn1 -- Ia_meas/LConn1
  Ia_meas/RConn1 -- Vab/LConn1
  B/RConn1 -- Vbc/LConn1 -- Vab/RConn1
  Vbc/RConn1 -- Ic_meas/RConn1

== system SSN_39busRT_Ctrl_4WT_19B/SM_master/4 WT/SS_windfarm1to2/Wind Farm (DFIG Type)/Wind Turbine Doubly-Fed Induction Generator (Average Model)1/Control System_average ==
  Vabc_B1 : Inport
  Q_ref : Inport  Port=2
  Iq_grid_conv_ref : Inport  Port=3
  wr : Inport  Port=4
  Iabc_grid_conv : Inport  Port=5
  Iabc_stator : Inport  Port=6
  Iabc_rotor : Inport  Port=7
  Q_B1 : Inport  Port=8
  angle_rotor : Inport  Port=9
  Vdc : Inport  Port=10
  Control : Subsystem
  Filter 1000 Hz : Subsystem  mask{Freq=1000, Zeta=0.707, Ts=Ts}
      mask prompts: Freq "Cut-off frequency (Hz):"; Zeta "Damping factor Zeta:"; Ts "Sample time"
  Unit Delay3 : UnitDelay  SampleTime=Ts  HasFrameUpgradeWarning=on
  Unit Delay4 : UnitDelay  SampleTime=Ts  HasFrameUpgradeWarning=on
  Uref_grid_conv : Outport
  Uref_rotor_conv : Outport  Port=2
  Theta_Freq : Outport  Port=3
  Pitch_angle : Outport  Port=4
  wires:
  wr/1 -> Filter 1000 Hz/9(wr)
  Q_B1/1 -> Filter 1000 Hz/8(Q_B1)
  Iabc_grid_conv/1 -> Filter 1000 Hz/2(Iabc_grid_conv)
  Iabc_rotor/1 -> Filter 1000 Hz/5(Iabc_rotor)
  Filter 1000 Hz/1("Vabc_B1 ") -> Control/1(Vabc_B1)
  Filter 1000 Hz/2("Iabc_grid_conv ") -> Control/2(Iabc_grid_conv)
  Filter 1000 Hz/3("Vdc ") -> Control/3(Vdc)
  Filter 1000 Hz/4("Iabc_stator ") -> Control/4(Iabc_stator)
  Filter 1000 Hz/5("Iabc_rotor ") -> Control/5(Iabc_rotor)
  Filter 1000 Hz/6("Q_ref ") -> Control/6(Q_ref)
  Filter 1000 Hz/7("Iq_grid_conv_ref ") -> Control/7(Iq_grid_conv_ref)
  Filter 1000 Hz/8("Q_B1 ") -> Control/8(Q_B1)
  Filter 1000 Hz/9("wr ") -> Control/9(wr)
  Filter 1000 Hz/10("angle_rotor ") -> Control/10(angle_rotor)
  Vabc_B1/1 -> Filter 1000 Hz/1(Vabc_B1)
  Iabc_stator/1 -> Filter 1000 Hz/4(Iabc_stator)
  Q_ref/1 -> Filter 1000 Hz/6(Q_ref)
  Iq_grid_conv_ref/1 -> Filter 1000 Hz/7(Iq_grid_conv_ref)
  Control/3(Theta_Freq) -> Theta_Freq/1
  Control/4(Pitch_angle) -> Pitch_angle/1
  Control/1(Uctrl_grid_conv) -> Unit Delay4/1
  Control/2(Uctrl_rotor_conv) -> Unit Delay3/1
  Vdc/1 -> Filter 1000 Hz/3(Vdc)
  angle_rotor/1 -> Filter 1000 Hz/10(angle_rotor)
  Unit Delay4/1 -> Uref_grid_conv/1
  Unit Delay3/1 -> Uref_rotor_conv/1

== system SSN_39busRT_Ctrl_4WT_19B/SM_master/4 WT/SS_windfarm1to2/Wind Farm (DFIG Type)/Wind Turbine Doubly-Fed Induction Generator (Average Model)1/Data acquisition electrical ==
  Vabc_B1 : Inport
  Iabc_B1 : Inport  Port=2
  Theta_Freq : Inport  Port=3
  Vdc : Inport  Port=4
  -->pu : Gain  Gain=1/(Pnom*NumberOfUnits)  SaturateOnIntegerOverflow=on  OutDataTypeStr=Inherit: Same as input  ParamDataTypeStr=Inherit: Same as input
  -1 : Gain  Gain=-1  SaturateOnIntegerOverflow=on  OutDataTypeStr=Inherit: Same as input  ParamDataTypeStr=Inherit: Same as input
  Bus Creator : BusCreator  Inputs=5
  Demux1 : Demux  Outputs=2
      settings: DisplayOption=none
  Demux2 : Demux  Outputs=2
      settings: DisplayOption=none
  Discrete 3-phase PLL-Driven Positive-Sequence Active & Reactive Power : powerlib_extras/Discrete Measurements/Discrete 3-phase PLL-Driven  Positive-Sequence Active & Reactive Power  Finit=Fnom  Fmin=45  Par_Vinit=[1 30]  Par_Iinit=[0.5 -10]  Ts=Ts_Control
      settings: SourceProductBaseCode=PS
  Mux : Mux  Inputs=2
  Terminator : Terminator
  Trigonometric Function : Trigonometry
  Trigonometric Function1 : Trigonometry  Operator=cos
  pu->A : Gain  Gain=Pnom*NumberOfUnits/sqrt(3)/Vnom*sqrt(2)  SaturateOnIntegerOverflow=on  OutDataTypeStr=Inherit: Same as input  ParamDataTypeStr=Inherit: Same as input
  pu->V : Gain  Gain=Vnom*sqrt(2)/sqrt(3)  SaturateOnIntegerOverflow=on  OutDataTypeStr=Inherit: Same as input  ParamDataTypeStr=Inherit: Same as input
  meas : Outport
  Q_B1 : Outport  Port=2
  wires:
  Demux2/2 -> Discrete 3-phase PLL-Driven Positive-Sequence Active & Reactive Power/1
  Demux2/1 -> Trigonometric Function1/1, Trigonometric Function/1
  Theta_Freq/1 -> Demux2/1
  Discrete 3-phase PLL-Driven Positive-Sequence Active & Reactive Power/1 -> Terminator/1
  Mux/1 -> Discrete 3-phase PLL-Driven Positive-Sequence Active & Reactive Power/2
  Trigonometric Function1/1 -> Mux/2
  Trigonometric Function/1 -> Mux/1
  pu->V/1 -> Discrete 3-phase PLL-Driven Positive-Sequence Active & Reactive Power/3
  Discrete 3-phase PLL-Driven Positive-Sequence Active & Reactive Power/2 -> -1/1
  pu->A/1 -> Discrete 3-phase PLL-Driven Positive-Sequence Active & Reactive Power/4
  Bus Creator/1 -> meas/1
  Iabc_B1/1 -> pu->A/1, Bus Creator/2  "Iabc_B1"
  Vabc_B1/1 -> pu->V/1, Bus Creator/1  "Vabc_B1"
  Vdc/1 -> Bus Creator/5  "Vdc"
  -1/1 -> Demux1/1
  Demux1/2 -> Bus Creator/4, -->pu/1  "Q_B1"
  Demux1/1 -> Bus Creator/3  "P_B1"
  -->pu/1 -> Q_B1/1

== system SSN_39busRT_Ctrl_4WT_19B/SM_master/4 WT/SS_windfarm1to2/Wind Farm (DFIG Type)/Wind Turbine Doubly-Fed Induction Generator (Average Model)1/Subsystem ==
  Current Measurement : spsCurrentMeasurementLib/Current Measurement  PhasorSimulation=off  OutputType=Complex  PSBequivalent=0
  Current Measurement1 : spsCurrentMeasurementLib/Current Measurement  PhasorSimulation=off  OutputType=Complex  PSBequivalent=0
  Current Measurement2 : spsCurrentMeasurementLib/Current Measurement  PhasorSimulation=off  OutputType=Complex  PSBequivalent=0
  Gain : Gain  Gain=1/(Pnom*NumberOfUnits/(Vnom*sqrt(3)))/sqrt(2)
  Mux : Mux  Inputs=3
  A : PMIOPort  Side=Left
  a : PMIOPort  Port=2  Side=Right
  B : PMIOPort  Port=3  Side=Left
  b : PMIOPort  Port=4  Side=Right
  C : PMIOPort  Port=5  Side=Left
  c : PMIOPort  Port=6  Side=Right
  IabcPU : Outport
  wires:
  Current Measurement2/1 -> Mux/3
  Current Measurement1/1 -> Mux/2
  Current Measurement/1 -> Mux/1
  Mux/1 -> Gain/1
  Gain/1 -> IabcPU/1
  connections:
  A/RConn1 -- Current Measurement/LConn1
  a/RConn1 -- Current Measurement/RConn1
  b/RConn1 -- Current Measurement1/RConn1
  B/RConn1 -- Current Measurement1/LConn1
  C/RConn1 -- Current Measurement2/LConn1
  c/RConn1 -- Current Measurement2/RConn1

== system SSN_39busRT_Ctrl_4WT_19B/SM_master/4 WT/SS_windfarm1to2/Wind Farm (DFIG Type)/Wind Turbine Doubly-Fed Induction Generator (Average Model)1/Subsystem1 ==
  Current Measurement : spsCurrentMeasurementLib/Current Measurement  PhasorSimulation=off  OutputType=Complex  PSBequivalent=0
  Current Measurement1 : spsCurrentMeasurementLib/Current Measurement  PhasorSimulation=off  OutputType=Complex  PSBequivalent=0
  Current Measurement2 : spsCurrentMeasurementLib/Current Measurement  PhasorSimulation=off  OutputType=Complex  PSBequivalent=0
  Gain : Gain  Gain=1/(Pnom*NumberOfUnits/(Vnom*sqrt(3)))/sqrt(2)
  Mux : Mux  Inputs=3
  A : PMIOPort  Side=Left
  a : PMIOPort  Port=2  Side=Right
  B : PMIOPort  Port=3  Side=Left
  b : PMIOPort  Port=4  Side=Right
  C : PMIOPort  Port=5  Side=Left
  c : PMIOPort  Port=6  Side=Right
  IabcPU : Outport
  wires:
  Gain/1 -> IabcPU/1
  Mux/1 -> Gain/1
  Current Measurement/1 -> Mux/1
  Current Measurement1/1 -> Mux/2
  Current Measurement2/1 -> Mux/3
  connections:
  c/RConn1 -- Current Measurement2/RConn1
  C/RConn1 -- Current Measurement2/LConn1
  B/RConn1 -- Current Measurement1/LConn1
  b/RConn1 -- Current Measurement1/RConn1
  a/RConn1 -- Current Measurement/RConn1
  A/RConn1 -- Current Measurement/LConn1

== system SSN_39busRT_Ctrl_4WT_19B/SM_master/4 WT/SS_windfarm1to2/Wind Farm (DFIG Type)/Wind Turbine Doubly-Fed Induction Generator (Average Model)1/Subsystem2 ==
  Current Measurement : spsCurrentMeasurementLib/Current Measurement  PhasorSimulation=off  OutputType=Complex  PSBequivalent=0
  Current Measurement1 : spsCurrentMeasurementLib/Current Measurement  PhasorSimulation=off  OutputType=Complex  PSBequivalent=0
  Current Measurement2 : spsCurrentMeasurementLib/Current Measurement  PhasorSimulation=off  OutputType=Complex  PSBequivalent=0
  Gain : Gain  Gain=1/(Pnom*NumberOfUnits/(Vnom*sqrt(3)))/sqrt(2)
  Mux : Mux  Inputs=3
  A : PMIOPort  Side=Left
  a : PMIOPort  Port=2  Side=Right
  B : PMIOPort  Port=3  Side=Left
  b : PMIOPort  Port=4  Side=Right
  C : PMIOPort  Port=5  Side=Left
  c : PMIOPort  Port=6  Side=Right
  IabcPU : Outport
  wires:
  Current Measurement2/1 -> Mux/3
  Current Measurement1/1 -> Mux/2
  Current Measurement/1 -> Mux/1
  Mux/1 -> Gain/1
  Gain/1 -> IabcPU/1
  connections:
  A/RConn1 -- Current Measurement/LConn1
  a/RConn1 -- Current Measurement/RConn1
  b/RConn1 -- Current Measurement1/RConn1
  B/RConn1 -- Current Measurement1/LConn1
  C/RConn1 -- Current Measurement2/LConn1
  c/RConn1 -- Current Measurement2/RConn1

== system SSN_39busRT_Ctrl_4WT_19B/SM_master/4 WT/SS_windfarm1to2/Wind Farm (DFIG Type)/Wind Turbine Doubly-Fed Induction Generator (Average Model)1/Wind Turbine v ==
  Generator speed (pu) : Inport
  Wind Power : Inport  Port=2
  Avoid division by zero : Saturate  UpperLimit=1e6  LowerLimit=1e-6
  Gain : Gain  Gain=-1  SaturateOnIntegerOverflow=on  OutDataTypeStr=Inherit: Same as input  ParamDataTypeStr=Inherit: Same as input
  Product2 : Product  Inputs=*/  InputSameDT=on  SaturateOnIntegerOverflow=on  OutDataTypeStr=Inherit: Same as first input
  pu->pu : Gain  Gain=P_wind_base*Pnom/Pelec_base  SaturateOnIntegerOverflow=on  OutDataTypeStr=Inherit: Same as input  ParamDataTypeStr=Inherit: Same as input
  Tm (pu) : Outport
  wires:
  Generator speed (pu)/1 -> Avoid division by zero/1
  pu->pu/1 -> Product2/1
  Gain/1 -> Tm (pu)/1
  Avoid division by zero/1 -> Product2/2
  Product2/1 -> Gain/1
  Wind Power/1 -> pu->pu/1

== system SSN_39busRT_Ctrl_4WT_19B/SM_master/4 WT/SS_windfarm1to2/Wind Farm (DFIG Type)1/Wind Turbine Doubly-Fed Induction Generator (Average Model)1/Average_VSC ==
  Uref : Inport
  Converter_model : Subsystem
  Demux : Demux  Outputs=2
  Ia_meas : spsCurrentMeasurementLib/Current Measurement  PhasorSimulation=off  OutputType=Complex  PSBequivalent=0
  Ic_meas : spsCurrentMeasurementLib/Current Measurement  PhasorSimulation=off  OutputType=Complex  PSBequivalent=0
  Idc : spsControlledCurrentSourceLib/Controlled Current Source  Initialize=on  Source_Type=AC  Amplitude=0  Phase=0  Frequency=0  Measurements=None
  Mux : Mux  Inputs=2
  Vab : spsControlledVoltageSourceLib/Controlled Voltage Source  Initialize=on  Source_Type=AC  Amplitude=0  Phase=0  Frequency=0  Measurements=None
  Vbc : spsControlledVoltageSourceLib/Controlled Voltage Source  Initialize=on  Source_Type=AC  Amplitude=0  Phase=0  Frequency=0  Measurements=None
  Vdc_meas : spsVoltageMeasurementLib/Voltage Measurement  PhasorSimulation=off  OutputType=Complex  PSBequivalent=0
  A : PMIOPort  Side=Left
  B : PMIOPort  Port=2  Side=Left
  C : PMIOPort  Port=3  Side=Left
  + : PMIOPort  Port=4  Side=Right
  - : PMIOPort  Port=5  Side=Right
  wires:
  Demux/2 -> Vbc/1  "Vbc"
  Demux/1 -> Vab/1  "Vab"
  Ia_meas/1 -> Mux/1  "Ia"
  Ic_meas/1 -> Mux/2  "Ic"
  Uref/1 -> Converter_model/3(Uref)
  Vdc_meas/1 -> Converter_model/2(Vdc)
  Mux/1 -> Converter_model/1(Ia_Ic)
  Converter_model/1(Idc) -> Idc/1  "Idc"
  Converter_model/2(Vab_Vbc) -> Demux/1
  connections:
  Vbc/RConn1 -- Ic_meas/RConn1
  Vab/RConn1 -- Vbc/LConn1 -- B/RConn1
  Ia_meas/RConn1 -- Vab/LConn1
  A/RConn1 -- Ia_meas/LConn1
  C/RConn1 -- Ic_meas/LConn1
  Vdc_meas/LConn2 -- +/RConn1 -- Idc/RConn1
  Vdc_meas/LConn1 -- -/RConn1 -- Idc/LConn1

== system SSN_39busRT_Ctrl_4WT_19B/SM_master/4 WT/SS_windfarm1to2/Wind Farm (DFIG Type)1/Wind Turbine Doubly-Fed Induction Generator (Average Model)1/Average_VSC1 ==
  Uref : Inport
  Converter_model : Subsystem
  Demux : Demux  Outputs=2
  Ia_meas : spsCurrentMeasurementLib/Current Measurement  PhasorSimulation=off  OutputType=Complex  PSBequivalent=0
  Ic_meas : spsCurrentMeasurementLib/Current Measurement  PhasorSimulation=off  OutputType=Complex  PSBequivalent=0
  Idc : spsControlledCurrentSourceLib/Controlled Current Source  Initialize=on  Source_Type=AC  Amplitude=0  Phase=0  Frequency=0  Measurements=None
  Mux : Mux  Inputs=2
  Vab : spsControlledVoltageSourceLib/Controlled Voltage Source  Initialize=on  Source_Type=AC  Amplitude=0  Phase=0  Frequency=0  Measurements=None
  Vbc : spsControlledVoltageSourceLib/Controlled Voltage Source  Initialize=on  Source_Type=AC  Amplitude=0  Phase=0  Frequency=0  Measurements=None
  Vdc_meas : spsVoltageMeasurementLib/Voltage Measurement  PhasorSimulation=off  OutputType=Complex  PSBequivalent=0
  A : PMIOPort  Side=Left
  B : PMIOPort  Port=2  Side=Left
  C : PMIOPort  Port=3  Side=Left
  + : PMIOPort  Port=4  Side=Right
  - : PMIOPort  Port=5  Side=Right
  wires:
  Demux/2 -> Vbc/1  "Vbc"
  Demux/1 -> Vab/1  "Vab"
  Ia_meas/1 -> Mux/1  "Ia"
  Ic_meas/1 -> Mux/2  "Ic"
  Uref/1 -> Converter_model/3(Uref)
  Vdc_meas/1 -> Converter_model/2(Vdc)
  Mux/1 -> Converter_model/1(Ia_Ic)
  Converter_model/1(Idc) -> Idc/1  "Idc"
  Converter_model/2(Vab_Vbc) -> Demux/1
  connections:
  Vbc/RConn1 -- Ic_meas/RConn1
  Vab/RConn1 -- Vbc/LConn1 -- B/RConn1
  Ia_meas/RConn1 -- Vab/LConn1
  A/RConn1 -- Ia_meas/LConn1
  C/RConn1 -- Ic_meas/LConn1
  Vdc_meas/LConn2 -- +/RConn1 -- Idc/RConn1
  Vdc_meas/LConn1 -- -/RConn1 -- Idc/LConn1

== system SSN_39busRT_Ctrl_4WT_19B/SM_master/4 WT/SS_windfarm1to2/Wind Farm (DFIG Type)1/Wind Turbine Doubly-Fed Induction Generator (Average Model)1/Control System_average ==
  Vabc_B1 : Inport
  Q_ref : Inport  Port=2
  Iq_grid_conv_ref : Inport  Port=3
  wr : Inport  Port=4
  Iabc_grid_conv : Inport  Port=5
  Iabc_stator : Inport  Port=6
  Iabc_rotor : Inport  Port=7
  Q_B1 : Inport  Port=8
  angle_rotor : Inport  Port=9
  Vdc : Inport  Port=10
  Control : Subsystem
  Filter 1000 Hz : Subsystem  mask{Freq=1000, Zeta=0.707, Ts=Ts}
      mask prompts: Freq "Cut-off frequency (Hz):"; Zeta "Damping factor Zeta:"; Ts "Sample time"
  Unit Delay3 : UnitDelay  SampleTime=Ts  HasFrameUpgradeWarning=on
  Unit Delay4 : UnitDelay  SampleTime=Ts  HasFrameUpgradeWarning=on
  Uref_grid_conv : Outport
  Uref_rotor_conv : Outport  Port=2
  Theta_Freq : Outport  Port=3
  Pitch_angle : Outport  Port=4
  wires:
  Unit Delay3/1 -> Uref_rotor_conv/1
  Unit Delay4/1 -> Uref_grid_conv/1
  angle_rotor/1 -> Filter 1000 Hz/10(angle_rotor)
  Vdc/1 -> Filter 1000 Hz/3(Vdc)
  Control/2(Uctrl_rotor_conv) -> Unit Delay3/1
  Control/1(Uctrl_grid_conv) -> Unit Delay4/1
  Control/4(Pitch_angle) -> Pitch_angle/1
  Control/3(Theta_Freq) -> Theta_Freq/1
  Iq_grid_conv_ref/1 -> Filter 1000 Hz/7(Iq_grid_conv_ref)
  Q_ref/1 -> Filter 1000 Hz/6(Q_ref)
  Iabc_stator/1 -> Filter 1000 Hz/4(Iabc_stator)
  Vabc_B1/1 -> Filter 1000 Hz/1(Vabc_B1)
  Filter 1000 Hz/10("angle_rotor ") -> Control/10(angle_rotor)
  Filter 1000 Hz/9("wr ") -> Control/9(wr)
  Filter 1000 Hz/8("Q_B1 ") -> Control/8(Q_B1)
  Filter 1000 Hz/7("Iq_grid_conv_ref ") -> Control/7(Iq_grid_conv_ref)
  Filter 1000 Hz/6("Q_ref ") -> Control/6(Q_ref)
  Filter 1000 Hz/5("Iabc_rotor ") -> Control/5(Iabc_rotor)
  Filter 1000 Hz/4("Iabc_stator ") -> Control/4(Iabc_stator)
  Filter 1000 Hz/3("Vdc ") -> Control/3(Vdc)
  Filter 1000 Hz/2("Iabc_grid_conv ") -> Control/2(Iabc_grid_conv)
  Filter 1000 Hz/1("Vabc_B1 ") -> Control/1(Vabc_B1)
  Iabc_rotor/1 -> Filter 1000 Hz/5(Iabc_rotor)
  Iabc_grid_conv/1 -> Filter 1000 Hz/2(Iabc_grid_conv)
  Q_B1/1 -> Filter 1000 Hz/8(Q_B1)
  wr/1 -> Filter 1000 Hz/9(wr)

== system SSN_39busRT_Ctrl_4WT_19B/SM_master/4 WT/SS_windfarm1to2/Wind Farm (DFIG Type)1/Wind Turbine Doubly-Fed Induction Generator (Average Model)1/Data acquisition electrical ==
  Vabc_B1 : Inport
  Iabc_B1 : Inport  Port=2
  Theta_Freq : Inport  Port=3
  Vdc : Inport  Port=4
  -->pu : Gain  Gain=1/(Pnom*NumberOfUnits)  SaturateOnIntegerOverflow=on  OutDataTypeStr=Inherit: Same as input  ParamDataTypeStr=Inherit: Same as input
  -1 : Gain  Gain=-1  SaturateOnIntegerOverflow=on  OutDataTypeStr=Inherit: Same as input  ParamDataTypeStr=Inherit: Same as input
  Bus Creator : BusCreator  Inputs=5
  Demux1 : Demux  Outputs=2
      settings: DisplayOption=none
  Demux2 : Demux  Outputs=2
      settings: DisplayOption=none
  Discrete 3-phase PLL-Driven Positive-Sequence Active & Reactive Power : powerlib_extras/Discrete Measurements/Discrete 3-phase PLL-Driven  Positive-Sequence Active & Reactive Power  Finit=Fnom  Fmin=45  Par_Vinit=[1 30]  Par_Iinit=[0.5 -10]  Ts=Ts_Control
      settings: SourceProductBaseCode=PS
  Mux : Mux  Inputs=2
  Terminator : Terminator
  Trigonometric Function : Trigonometry
  Trigonometric Function1 : Trigonometry  Operator=cos
  pu->A : Gain  Gain=Pnom*NumberOfUnits/sqrt(3)/Vnom*sqrt(2)  SaturateOnIntegerOverflow=on  OutDataTypeStr=Inherit: Same as input  ParamDataTypeStr=Inherit: Same as input
  pu->V : Gain  Gain=Vnom*sqrt(2)/sqrt(3)  SaturateOnIntegerOverflow=on  OutDataTypeStr=Inherit: Same as input  ParamDataTypeStr=Inherit: Same as input
  meas : Outport
  Q_B1 : Outport  Port=2
  wires:
  -->pu/1 -> Q_B1/1
  Demux1/1 -> Bus Creator/3  "P_B1"
  Demux1/2 -> -->pu/1, Bus Creator/4  "Q_B1"
  -1/1 -> Demux1/1
  Vdc/1 -> Bus Creator/5  "Vdc"
  Vabc_B1/1 -> Bus Creator/1, pu->V/1  "Vabc_B1"
  Iabc_B1/1 -> Bus Creator/2, pu->A/1  "Iabc_B1"
  Bus Creator/1 -> meas/1
  pu->A/1 -> Discrete 3-phase PLL-Driven Positive-Sequence Active & Reactive Power/4
  Discrete 3-phase PLL-Driven Positive-Sequence Active & Reactive Power/2 -> -1/1
  pu->V/1 -> Discrete 3-phase PLL-Driven Positive-Sequence Active & Reactive Power/3
  Trigonometric Function/1 -> Mux/1
  Trigonometric Function1/1 -> Mux/2
  Mux/1 -> Discrete 3-phase PLL-Driven Positive-Sequence Active & Reactive Power/2
  Discrete 3-phase PLL-Driven Positive-Sequence Active & Reactive Power/1 -> Terminator/1
  Theta_Freq/1 -> Demux2/1
  Demux2/1 -> Trigonometric Function/1, Trigonometric Function1/1
  Demux2/2 -> Discrete 3-phase PLL-Driven Positive-Sequence Active & Reactive Power/1

== system SSN_39busRT_Ctrl_4WT_19B/SM_master/4 WT/SS_windfarm1to2/Wind Farm (DFIG Type)1/Wind Turbine Doubly-Fed Induction Generator (Average Model)1/Subsystem ==
  Current Measurement : spsCurrentMeasurementLib/Current Measurement  PhasorSimulation=off  OutputType=Complex  PSBequivalent=0
  Current Measurement1 : spsCurrentMeasurementLib/Current Measurement  PhasorSimulation=off  OutputType=Complex  PSBequivalent=0
  Current Measurement2 : spsCurrentMeasurementLib/Current Measurement  PhasorSimulation=off  OutputType=Complex  PSBequivalent=0
  Gain : Gain  Gain=1/(Pnom*NumberOfUnits/(Vnom*sqrt(3)))/sqrt(2)
  Mux : Mux  Inputs=3
  A : PMIOPort  Side=Left
  a : PMIOPort  Port=2  Side=Right
  B : PMIOPort  Port=3  Side=Left
  b : PMIOPort  Port=4  Side=Right
  C : PMIOPort  Port=5  Side=Left
  c : PMIOPort  Port=6  Side=Right
  IabcPU : Outport
  wires:
  Gain/1 -> IabcPU/1
  Mux/1 -> Gain/1
  Current Measurement/1 -> Mux/1
  Current Measurement1/1 -> Mux/2
  Current Measurement2/1 -> Mux/3
  connections:
  c/RConn1 -- Current Measurement2/RConn1
  C/RConn1 -- Current Measurement2/LConn1
  B/RConn1 -- Current Measurement1/LConn1
  b/RConn1 -- Current Measurement1/RConn1
  a/RConn1 -- Current Measurement/RConn1
  A/RConn1 -- Current Measurement/LConn1

== system SSN_39busRT_Ctrl_4WT_19B/SM_master/4 WT/SS_windfarm1to2/Wind Farm (DFIG Type)1/Wind Turbine Doubly-Fed Induction Generator (Average Model)1/Subsystem1 ==
  Current Measurement : spsCurrentMeasurementLib/Current Measurement  PhasorSimulation=off  OutputType=Complex  PSBequivalent=0
  Current Measurement1 : spsCurrentMeasurementLib/Current Measurement  PhasorSimulation=off  OutputType=Complex  PSBequivalent=0
  Current Measurement2 : spsCurrentMeasurementLib/Current Measurement  PhasorSimulation=off  OutputType=Complex  PSBequivalent=0
  Gain : Gain  Gain=1/(Pnom*NumberOfUnits/(Vnom*sqrt(3)))/sqrt(2)
  Mux : Mux  Inputs=3
  A : PMIOPort  Side=Left
  a : PMIOPort  Port=2  Side=Right
  B : PMIOPort  Port=3  Side=Left
  b : PMIOPort  Port=4  Side=Right
  C : PMIOPort  Port=5  Side=Left
  c : PMIOPort  Port=6  Side=Right
  IabcPU : Outport
  wires:
  Current Measurement2/1 -> Mux/3
  Current Measurement1/1 -> Mux/2
  Current Measurement/1 -> Mux/1
  Mux/1 -> Gain/1
  Gain/1 -> IabcPU/1
  connections:
  A/RConn1 -- Current Measurement/LConn1
  a/RConn1 -- Current Measurement/RConn1
  b/RConn1 -- Current Measurement1/RConn1
  B/RConn1 -- Current Measurement1/LConn1
  C/RConn1 -- Current Measurement2/LConn1
  c/RConn1 -- Current Measurement2/RConn1

== system SSN_39busRT_Ctrl_4WT_19B/SM_master/4 WT/SS_windfarm1to2/Wind Farm (DFIG Type)1/Wind Turbine Doubly-Fed Induction Generator (Average Model)1/Subsystem2 ==
  Current Measurement : spsCurrentMeasurementLib/Current Measurement  PhasorSimulation=off  OutputType=Complex  PSBequivalent=0
  Current Measurement1 : spsCurrentMeasurementLib/Current Measurement  PhasorSimulation=off  OutputType=Complex  PSBequivalent=0
  Current Measurement2 : spsCurrentMeasurementLib/Current Measurement  PhasorSimulation=off  OutputType=Complex  PSBequivalent=0
  Gain : Gain  Gain=1/(Pnom*NumberOfUnits/(Vnom*sqrt(3)))/sqrt(2)
  Mux : Mux  Inputs=3
  A : PMIOPort  Side=Left
  a : PMIOPort  Port=2  Side=Right
  B : PMIOPort  Port=3  Side=Left
  b : PMIOPort  Port=4  Side=Right
  C : PMIOPort  Port=5  Side=Left
  c : PMIOPort  Port=6  Side=Right
  IabcPU : Outport
  wires:
  Gain/1 -> IabcPU/1
  Mux/1 -> Gain/1
  Current Measurement/1 -> Mux/1
  Current Measurement1/1 -> Mux/2
  Current Measurement2/1 -> Mux/3
  connections:
  c/RConn1 -- Current Measurement2/RConn1
  C/RConn1 -- Current Measurement2/LConn1
  B/RConn1 -- Current Measurement1/LConn1
  b/RConn1 -- Current Measurement1/RConn1
  a/RConn1 -- Current Measurement/RConn1
  A/RConn1 -- Current Measurement/LConn1

== system SSN_39busRT_Ctrl_4WT_19B/SM_master/4 WT/SS_windfarm1to2/Wind Farm (DFIG Type)1/Wind Turbine Doubly-Fed Induction Generator (Average Model)1/Wind Turbine v ==
  Generator speed (pu) : Inport
  Wind Power : Inport  Port=2
  Avoid division by zero : Saturate  UpperLimit=1e6  LowerLimit=1e-6
  Gain : Gain  Gain=-1  SaturateOnIntegerOverflow=on  OutDataTypeStr=Inherit: Same as input  ParamDataTypeStr=Inherit: Same as input
  Product2 : Product  Inputs=*/  InputSameDT=on  SaturateOnIntegerOverflow=on  OutDataTypeStr=Inherit: Same as first input
  pu->pu : Gain  Gain=P_wind_base*Pnom/Pelec_base  SaturateOnIntegerOverflow=on  OutDataTypeStr=Inherit: Same as input  ParamDataTypeStr=Inherit: Same as input
  Tm (pu) : Outport
  wires:
  Product2/1 -> Gain/1
  Avoid division by zero/1 -> Product2/2
  Gain/1 -> Tm (pu)/1
  pu->pu/1 -> Product2/1
  Generator speed (pu)/1 -> Avoid division by zero/1
  Wind Power/1 -> pu->pu/1
